simulink model "Phasor_load"  (R2024a)
settings: Solver=ode1  StartTime=0.0  StopTime=simtime  FixedStep=Ts  RelTol=1e-3
values from neighbouring files (symbols this model uses):
  c0 = c0_hawk    (= 6.37282e-09)    [EMT_Phasor_parameters.m]
  c1 = c1_hawk    (= 8.76156e-09)    [EMT_Phasor_parameters.m]
  fg = 50    [EMT_Phasor_parameters.m]
  G1gen = 0.1245    [EMT_Phasor_parameters.m]
  G2gen = 0.30    (= 0.3)    [EMT_Phasor_parameters.m]
  G3gen = 0.20    (= 0.2)    [EMT_Phasor_parameters.m]
  G4sgen = 0.2078    [EMT_Phasor_parameters.m]
  G5gen = 0.20    (= 0.2)    [EMT_Phasor_parameters.m]
  G6gen = 0.2078    [EMT_Phasor_parameters.m]
  G6sgen = 0.20    (= 0.2)    [EMT_Phasor_parameters.m]
  G7gen = 0.518    [EMT_Phasor_parameters.m]
  Ihvpk = Ihv*sqrt(2)    [EMT_Phasor_parameters.m]
  l0 = l0_hawk    (= 0.00373)    [EMT_Phasor_parameters.m]
  l1 = l1_hawk    (= 0.00133)    [EMT_Phasor_parameters.m]
  L3dem = 0.10    (= 0.1)    [EMT_Phasor_parameters.m]
  L4dem = 0.30    (= 0.3)    [EMT_Phasor_parameters.m]
  L5dem = 0.35    [EMT_Phasor_parameters.m]
  L6dem = 0.15    [EMT_Phasor_parameters.m]
  L7dem = 0.10    (= 0.1)    [EMT_Phasor_parameters.m]
  Pr = Sr*PF    (= 550050000)    [EMT_Phasor_parameters.m]
  Qr = sqrt(Sr^2 - Pr^2)    [EMT_Phasor_parameters.m]
  r0 = r0_hawk    (= 0.44587)    [EMT_Phasor_parameters.m]
  r1 = r1_hawk    (= 0.12087)    [EMT_Phasor_parameters.m]
  Rtpu = Xtpu/40    (= 0.00375)    [EMT_Phasor_parameters.m]
  S1non = 400e6    (= 400000000)    [EMT_Phasor_parameters.m]
  S2non = 300e6    (= 300000000)    [EMT_Phasor_parameters.m]
  S3non = 200e6    (= 200000000)    [EMT_Phasor_parameters.m]
  S4snon = 200e6    (= 200000000)    [EMT_Phasor_parameters.m]
  S5non = 500e6    (= 500000000)    [EMT_Phasor_parameters.m]
  S6non = 400e6    (= 400000000)    [EMT_Phasor_parameters.m]
  S6snon = 200e6    (= 200000000)    [EMT_Phasor_parameters.m]
  S7non = 200e6    (= 200000000)    [EMT_Phasor_parameters.m]
  simtime = 5    [EMT_Phasor_parameters.m]
  tonvsc = 0.01    [EMT_Phasor_parameters.m]
  Ts = 150e-6    (= 0.00015)    [EMT_Phasor_parameters.m]
  Vhv = 220e3    (= 220000)    [EMT_Phasor_parameters.m]
  Vmv = 22e3    (= 22000)    [EMT_Phasor_parameters.m]
  wc1 = wsw1/10    (= 848.230016469)    [EMT_Phasor_parameters.m]
  wdc1 = wc1/10    (= 84.8230016469)    [EMT_Phasor_parameters.m]
  wpq1 = wc1/10    (= 84.8230016469)    [EMT_Phasor_parameters.m]
  wsw1 = ksw1*2*pi*fg    (= 8482.30016469)    [EMT_Phasor_parameters.m]
  Xtpu = 0.15    [EMT_Phasor_parameters.m]
undefined symbols (not defined in the file or in its folder): D11, Delta, Kf, r, theta0
libraries: simulink_extras x152, spsGroundLib x52, powerlib_meascontrol x52, pid_lib x40, spsCurrentMeasurementLib x39, spsVoltageMeasurementLib x33, simulink x32, eeGeneralControl x32, eeTransforms x24, powerlib x24, spsFirstOrderFilterLib x16, spsControlledCurrentSourceLib x12
(part 16 of 17)

== system Phasor_load/G6/VSC/VSC Control/Modulation/Phasor Quasi-EMT/V to I RL (+seq) ==
  note: d-q axis model of a 3-phase series R-L branch
  note: Using Laplace transform:
  note: Iq = (Vq1 - Vq2 - w*L*Id)/(R + s*L)
  note: Id = (Vd1 - Vd2 + w*L*Iq)/(R + s*L)
  note: V2
  note: ==========================================================================================
  note: V1
  note: Vq1 - Vq2 = [ R * Iq ] + [ L* w * Id ] + [ L * d/dt (Iq) ]
  note: where w = 2*pi*f
  note: I --->
  note: o--------| R |---| L |-------o
  note: Vd1 - Vd2 = [ R * Id ] - [ L* w * Iq ] + [ L * d/dt (Id) ]
  note: This subsystem converts the VSC output voltage in a current signal through an RL element
  Vdq1 : Inport
  Vdq2 : Inport  Port=2
  Cartesian to Polar : simulink_extras/Transformations/Cartesian to Polar
  Delay : Delay  DelayLength=1
  Demux : Demux  Outputs=2
  Mux : Mux  Inputs=2
  Polar to Cartesian : simulink_extras/Transformations/Polar to Cartesian
  R_choke1 : Gain  Gain=w*L  SaturateOnIntegerOverflow=on  OutDataTypeStr=Inherit: Same as input  ParamDataTypeStr=Inherit: Same as input
  R_choke2 : Gain  Gain=[1 -1]  SaturateOnIntegerOverflow=on  OutDataTypeStr=Inherit: Same as input  ParamDataTypeStr=Inherit: Same as input
  Saturation : Saturate  UpperLimit=Imax  LowerLimit=0
  Selector : Selector  InputPortWidth=2  IndexOptions=Index vector (dialog)  Indices=[2 1]  OutputSizes=1
  Sum : Sum  Inputs=+-+  SaturateOnIntegerOverflow=on
  Transfer Fcn (with initial outputs) : simulink_extras/Additional Linear/Transfer Fcn (with initial outputs)  N=[1]  D=[L R]  Y0=0  U0=0
  Transfer Fcn (with initial outputs)1 : simulink_extras/Additional Linear/Transfer Fcn (with initial outputs)  N=[1]  D=[L R]  Y0=0  U0=0
  idIq : Outport  VectorParamsAs1DForOutWhenUnconnected=off
  wires:
  Selector/1 -> R_choke1/1
  Vdq1/1 -> Sum/1
  R_choke1/1 -> R_choke2/1
  Sum/1 -> Demux/1
  Demux/1 -> Transfer Fcn (with initial outputs)/1
  Demux/2 -> Transfer Fcn (with initial outputs)1/1
  Polar to Cartesian/1 -> Mux/1
  Polar to Cartesian/2 -> Mux/2
  Cartesian to Polar/2 -> Polar to Cartesian/2
  Mux/1 -> Delay/1, idIq/1
  R_choke2/1 -> Sum/3
  Transfer Fcn (with initial outputs)/1 -> Cartesian to Polar/1
  Transfer Fcn (with initial outputs)1/1 -> Cartesian to Polar/2
  Vdq2/1 -> Sum/2
  Cartesian to Polar/1 -> Saturation/1
  Saturation/1 -> Polar to Cartesian/1
  Delay/1 -> Selector/1

== system Phasor_load/G6/VSC/VSC Control/Modulation/Phasor Quasi-EMT/V to I RL (- seq) ==
  note: d-q axis model of a 3-phase series R-L branch
  note: Using Laplace transform:
  note: Iq = (Vq1 - Vq2 - w*L*Id)/(R + s*L)
  note: Id = (Vd1 - Vd2 + w*L*Iq)/(R + s*L)
  note: V2
  note: ==========================================================================================
  note: V1
  note: Vq1 - Vq2 = [ R * Iq ] + [ L* w * Id ] + [ L * d/dt (Iq) ]
  note: where w = 2*pi*f
  note: I --->
  note: o--------| R |---| L |-------o
  note: Vd1 - Vd2 = [ R * Id ] - [ L* w * Iq ] + [ L * d/dt (Id) ]
  note: This subsystem converts the VSC output voltage in a current signal through an RL element
  Vdq1 : Inport
  Vdq2 : Inport  Port=2
  Cartesian to Polar : simulink_extras/Transformations/Cartesian to Polar
  Delay : Delay  DelayLength=1
  Demux : Demux  Outputs=2
  Mux : Mux  Inputs=2
  Polar to Cartesian : simulink_extras/Transformations/Polar to Cartesian
  R_choke1 : Gain  Gain=w*L  SaturateOnIntegerOverflow=on  OutDataTypeStr=Inherit: Same as input  ParamDataTypeStr=Inherit: Same as input
  R_choke2 : Gain  Gain=[-1 1]  SaturateOnIntegerOverflow=on  OutDataTypeStr=Inherit: Same as input  ParamDataTypeStr=Inherit: Same as input
  Saturation : Saturate  UpperLimit=Imax  LowerLimit=0
  Selector : Selector  InputPortWidth=2  IndexOptions=Index vector (dialog)  Indices=[2 1]  OutputSizes=1
  Sum : Sum  Inputs=+-+  SaturateOnIntegerOverflow=on
  Transfer Fcn (with initial outputs) : simulink_extras/Additional Linear/Transfer Fcn (with initial outputs)  N=[1]  D=[L R]  Y0=0  U0=0
  Transfer Fcn (with initial outputs)1 : simulink_extras/Additional Linear/Transfer Fcn (with initial outputs)  N=[1]  D=[L R]  Y0=0  U0=0
  idIq : Outport  VectorParamsAs1DForOutWhenUnconnected=off
  wires:
  Selector/1 -> R_choke1/1
  Vdq1/1 -> Sum/1
  R_choke1/1 -> R_choke2/1
  Sum/1 -> Demux/1
  Demux/1 -> Transfer Fcn (with initial outputs)/1
  Demux/2 -> Transfer Fcn (with initial outputs)1/1
  Polar to Cartesian/1 -> Mux/1
  Polar to Cartesian/2 -> Mux/2
  Cartesian to Polar/2 -> Polar to Cartesian/2
  Mux/1 -> Delay/1, idIq/1
  R_choke2/1 -> Sum/3
  Transfer Fcn (with initial outputs)/1 -> Cartesian to Polar/1
  Transfer Fcn (with initial outputs)1/1 -> Cartesian to Polar/2
  Vdq2/1 -> Sum/2
  Cartesian to Polar/1 -> Saturation/1
  Saturation/1 -> Polar to Cartesian/1
  Delay/1 -> Selector/1

== system Phasor_load/G2/VSC/VSC Control/Control loops/Phasor I 1st/Outer-loop/Power calculation ==
  note: AC power calculation using symmetrical components in dq axis
  note: Pavgp = 3/2*(vqp*iqp + vdp*idp) and Qavgp = 3/2*(vqp*idp-vdp*iqp)
  note: P = Pavg + Pc2*cos(2wt) + Ps2*sin(2wt) ---> Pavg = Pavgp + Pavgn
  note: Q = Qavg + Qc2*cos(2wt) + Qs2*sin(2wt) ---> Qavg = Qavgp + Qavgn
  note: Pavgn = 3/2*(vqn*iqn + vdn*idn) and Qavgn = 3/2*(vqn*idn-vdn*iqn)
  vq+ : Inport
  vd+ : Inport  Port=2
  iq+ : Inport  Port=3
  id+ : Inport  Port=4
  vq- : Inport  Port=5
  vd- : Inport  Port=6
  iq- : Inport  Port=7
  id- : Inport  Port=8
  Gain : Gain  Gain=3/2
  Gain1 : Gain  Gain=3/2
  Gain2 : Gain  Gain=-1
  Gain3 : Gain  Gain=-1
  Mux{,1..3} (4 alike) : Mux  Inputs=2
  Product{,1..3} (4 alike) : Product
  Sum1 : Sum
  Sum2 : Sum
  Sum8 : Sum
  PQ : Outport
  wires:
  Sum8/1 -> Gain/1
  Gain2/1 -> Mux2/2
  Mux2/1 -> Product2/2
  Product2/1 -> Sum8/2
  Mux/1 -> Product/2
  Product/1 -> Sum8/1
  iq+/1 -> [iqp]
  [iqp] -> Gain2/1, Mux/1
  id+/1 -> [idp]
  [idp] -> Mux2/1, Mux/2
  vq+/1 -> [vqp]
  [vqp] -> Product/1
  vd+/1 -> [vdp]
  [vdp] -> Product2/1
  Gain/1 -> Sum1/1
  Sum1/1 -> PQ/1
  Gain3/1 -> Mux3/2
  Mux1/1 -> Product1/2
  Product3/1 -> Sum2/2
  Product1/1 -> Sum2/1
  [vdn] -> Product3/1
  Mux3/1 -> Product3/2
  [vqn] -> Product1/1
  Sum2/1 -> Gain1/1
  [iqn] -> Gain3/1, Mux1/1
  [idn] -> Mux3/1, Mux1/2
  vq-/1 -> [vqn]
  vd-/1 -> [vdn]
  iq-/1 -> [iqn]
  id-/1 -> [idn]
  Gain1/1 -> Sum1/2

== system Phasor_load/G2/VSC/VSC Control/Control loops/Phasor I ref/Outer-loop/Power calculation ==
  note: Pavgn = 3/2*(vqn*iqn + vdn*idn) and Qavgn = 3/2*(vqn*idn-vdn*iqn)
  note: Q = Qavg + Qc2*cos(2wt) + Qs2*sin(2wt) ---> Qavg = Qavgp + Qavgn
  note: P = Pavg + Pc2*cos(2wt) + Ps2*sin(2wt) ---> Pavg = Pavgp + Pavgn
  note: Pavgp = 3/2*(vqp*iqp + vdp*idp) and Qavgp = 3/2*(vqp*idp-vdp*iqp)
  note: AC power calculation using symmetrical components in dq axis
  vq+ : Inport
  vd+ : Inport  Port=2
  iq+ : Inport  Port=3
  id+ : Inport  Port=4
  vq- : Inport  Port=5
  vd- : Inport  Port=6
  iq- : Inport  Port=7
  id- : Inport  Port=8
  Gain : Gain  Gain=3/2
  Gain1 : Gain  Gain=3/2
  Gain2 : Gain  Gain=-1
  Gain3 : Gain  Gain=-1
  Mux{,1..3} (4 alike) : Mux  Inputs=2
  Product{,1..3} (4 alike) : Product
  Sum1 : Sum
  Sum2 : Sum
  Sum8 : Sum
  PQ : Outport
  wires:
  Gain1/1 -> Sum1/2
  id-/1 -> [idn]
  iq-/1 -> [iqn]
  vd-/1 -> [vdn]
  vq-/1 -> [vqn]
  [idn] -> Mux1/2, Mux3/1
  [iqn] -> Mux1/1, Gain3/1
  Sum2/1 -> Gain1/1
  [vqn] -> Product1/1
  Mux3/1 -> Product3/2
  [vdn] -> Product3/1
  Product1/1 -> Sum2/1
  Product3/1 -> Sum2/2
  Mux1/1 -> Product1/2
  Gain3/1 -> Mux3/2
  Sum1/1 -> PQ/1
  Gain/1 -> Sum1/1
  [vdp] -> Product2/1
  vd+/1 -> [vdp]
  [vqp] -> Product/1
  vq+/1 -> [vqp]
  [idp] -> Mux/2, Mux2/1
  id+/1 -> [idp]
  [iqp] -> Mux/1, Gain2/1
  iq+/1 -> [iqp]
  Product/1 -> Sum8/1
  Mux/1 -> Product/2
  Product2/1 -> Sum8/2
  Mux2/1 -> Product2/2
  Gain2/1 -> Mux2/2
  Sum8/1 -> Gain/1

== system Phasor_load/G2/VSC/VSC Control/Control loops/Phasor PQ 1st/Outer-loop/Power calculation ==
  note: AC power calculation using symmetrical components in dq axis
  note: Pavgp = 3/2*(vqp*iqp + vdp*idp) and Qavgp = 3/2*(vqp*idp-vdp*iqp)
  note: P = Pavg + Pc2*cos(2wt) + Ps2*sin(2wt) ---> Pavg = Pavgp + Pavgn
  note: Q = Qavg + Qc2*cos(2wt) + Qs2*sin(2wt) ---> Qavg = Qavgp + Qavgn
  note: Pavgn = 3/2*(vqn*iqn + vdn*idn) and Qavgn = 3/2*(vqn*idn-vdn*iqn)
  vq+ : Inport
  vd+ : Inport  Port=2
  iq+ : Inport  Port=3
  id+ : Inport  Port=4
  vq- : Inport  Port=5
  vd- : Inport  Port=6
  iq- : Inport  Port=7
  id- : Inport  Port=8
  Gain : Gain  Gain=3/2
  Gain1 : Gain  Gain=3/2
  Gain2 : Gain  Gain=-1
  Gain3 : Gain  Gain=-1
  Mux{,1..3} (4 alike) : Mux  Inputs=2
  Product{,1..3} (4 alike) : Product
  Sum1 : Sum
  Sum2 : Sum
  Sum8 : Sum
  PQ : Outport
  wires:
  Sum8/1 -> Gain/1
  Gain2/1 -> Mux2/2
  Mux2/1 -> Product2/2
  Product2/1 -> Sum8/2
  Mux/1 -> Product/2
  Product/1 -> Sum8/1
  iq+/1 -> [iqp]
  [iqp] -> Gain2/1, Mux/1
  id+/1 -> [idp]
  [idp] -> Mux2/1, Mux/2
  vq+/1 -> [vqp]
  [vqp] -> Product/1
  vd+/1 -> [vdp]
  [vdp] -> Product2/1
  Gain/1 -> Sum1/1
  Sum1/1 -> PQ/1
  Gain3/1 -> Mux3/2
  Mux1/1 -> Product1/2
  Product3/1 -> Sum2/2
  Product1/1 -> Sum2/1
  [vdn] -> Product3/1
  Mux3/1 -> Product3/2
  [vqn] -> Product1/1
  Sum2/1 -> Gain1/1
  [iqn] -> Gain3/1, Mux1/1
  [idn] -> Mux3/1, Mux1/2
  vq-/1 -> [vqn]
  vd-/1 -> [vdn]
  iq-/1 -> [iqn]
  id-/1 -> [idn]
  Gain1/1 -> Sum1/2

== system Phasor_load/G2/VSC/VSC Control/Control loops/SW, EMT AVG, Phasor Quasi-EMT/Outer-loop/Power calculation ==
  note: AC power calculation using symmetrical components in dq axis
  note: Pavgp = 3/2*(vqp*iqp + vdp*idp) and Qavgp = 3/2*(vqp*idp-vdp*iqp)
  note: P = Pavg + Pc2*cos(2wt) + Ps2*sin(2wt) ---> Pavg = Pavgp + Pavgn
  note: Q = Qavg + Qc2*cos(2wt) + Qs2*sin(2wt) ---> Qavg = Qavgp + Qavgn
  note: Pavgn = 3/2*(vqn*iqn + vdn*idn) and Qavgn = 3/2*(vqn*idn-vdn*iqn)
  vq+ : Inport
  vd+ : Inport  Port=2
  iq+ : Inport  Port=3
  id+ : Inport  Port=4
  vq- : Inport  Port=5
  vd- : Inport  Port=6
  iq- : Inport  Port=7
  id- : Inport  Port=8
  Gain : Gain  Gain=3/2
  Gain1 : Gain  Gain=3/2
  Gain2 : Gain  Gain=-1
  Gain3 : Gain  Gain=-1
  Mux{,1..3} (4 alike) : Mux  Inputs=2
  Product{,1..3} (4 alike) : Product
  Sum1 : Sum
  Sum2 : Sum
  Sum8 : Sum
  PQ : Outport
  wires:
  Sum8/1 -> Gain/1
  Gain2/1 -> Mux2/2
  Mux2/1 -> Product2/2
  Product2/1 -> Sum8/2
  Mux/1 -> Product/2
  Product/1 -> Sum8/1
  iq+/1 -> [iqp]
  [iqp] -> Gain2/1, Mux/1
  id+/1 -> [idp]
  [idp] -> Mux2/1, Mux/2
  vq+/1 -> [vqp]
  [vqp] -> Product/1
  vd+/1 -> [vdp]
  [vdp] -> Product2/1
  Gain/1 -> Sum1/1
  Sum1/1 -> PQ/1
  Gain3/1 -> Mux3/2
  Mux1/1 -> Product1/2
  Product3/1 -> Sum2/2
  Product1/1 -> Sum2/1
  [vdn] -> Product3/1
  Mux3/1 -> Product3/2
  [vqn] -> Product1/1
  Sum2/1 -> Gain1/1
  [iqn] -> Gain3/1, Mux1/1
  [idn] -> Mux3/1, Mux1/2
  vq-/1 -> [vqn]
  vd-/1 -> [vdn]
  iq-/1 -> [iqn]
  id-/1 -> [idn]
  Gain1/1 -> Sum1/2

== system Phasor_load/G2/VSC/VSC Control/Measurements/EMT/PLL aligned with positive-sequence/Notch filter ==
  In : Inport
  Discrete Transfer Fcn : DiscreteTransferFcn  Numerator=[1, -2*cos(theta0), 1]  Denominator="[1, -2*cos(theta0)*r,  r^2]"
  Gain7 : Gain  Gain=Kf
  Out : Outport
  wires:
  Gain7/1 -> Discrete Transfer Fcn/1
  Discrete Transfer Fcn/1 -> Out/1
  In/1 -> Gain7/1

== system Phasor_load/G2/VSC/VSC Control/Measurements/EMT/PLL aligned with positive-sequence/Park transform ==
  note: Park transform (q axis leading)
  abc : Inport
  theta : Inport  Port=2
  0 : Fcn  Expr=1/3*(u(1) + u(2) + u(3))
  Mux2 : Mux  Inputs=2
  Mux3 : Mux  Inputs=3
  d : Fcn  Expr=2/3*(u(1)*sin(u(4)) + u(2)*sin(u(4) - (2*pi)/3) + u(3)*sin(u(4) + (2*pi)/3))
  q : Fcn  Expr=2/3*(u(1)*cos(u(4)) + u(2)*cos(u(4) - (2*pi)/3) + u(3)*cos(u(4) + (2*pi)/3))
  qd0 : Outport  VectorParamsAs1DForOutWhenUnconnected=off
  wires:
  q/1 -> Mux3/1
  Mux2/1 -> q/1, 0/1, d/1
  0/1 -> Mux3/3
  d/1 -> Mux3/2
  theta/1 -> Mux2/2
  abc/1 -> Mux2/1
  Mux3/1 -> qd0/1

== system Phasor_load/G2/VSC/VSC Control/Measurements/EMT/PLL aligned with positive-sequence/Phase-sequence separation ==
  note: Phase-sequence separation based on
      | Delayed Signal Cancellation (DSC) method
  abc : Inport
  Theta : Inport  Port=2
  Complex to Real-Imag1 : ComplexToRealImag
  Complex to Real-Imag2 : ComplexToRealImag
  Complex to Real-Imag3 : ComplexToRealImag
  Constant : Constant  Value=negseq_en
  Demux3 : Demux  Outputs=3
  Exp2 : Math  OutputSignalType=complex
  Exp3 : Math  OutputSignalType=complex
  Gain1 : Gain  Gain=1/2
  Gain4 : Gain  Gain=-1i
  Gain5 : Gain  Gain=1i
  Gain6 : Gain  Gain=1/2
  Gain7 : Gain  Gain=1i
  NOT : Logic  Operator=NOT  IconShape=distinctive  AllPortsSameDT=off  OutDataTypeStr=boolean
  Product3 : Product
  Product4 : Product
  Real-Imag to Complex : RealImagToComplex
  Real-Imag to Complex1 : RealImagToComplex
  Sum1 : Sum  Inputs=|++
  Sum2 : Sum  Inputs=-+|
  Switch : Switch  Criteria=u2 ~= 0  SaturateOnIntegerOverflow=off  InputSameDT=off
  Terminator3 : Terminator
  Transport Delay2 : TransportDelay  DelayTime=1/4*(1/50)
  Transport Delay3 : TransportDelay  DelayTime=1/4*(1/50)
  abc to Alpha-Beta-Zero : powerlib_meascontrol/Transformations/abc to Alpha-Beta-Zero
  q+ : Outport
  d+ : Outport  Port=2
  q- : Outport  Port=3
  d- : Outport  Port=4
  wires:
  NOT/1 -> Switch/2
  Constant/1 -> NOT/1
  Switch/1 -> Product3/1
  Gain6/1 -> Switch/3
  Sum2/1 -> Gain1/1
  Transport Delay2/1 -> Real-Imag to Complex1/1
  Demux3/1 -> Real-Imag to Complex/1
  Complex to Real-Imag1/2 -> Transport Delay3/1
  Gain1/1 -> Product4/2
  Real-Imag to Complex/1 -> Complex to Real-Imag1/1, Sum2/2, Sum1/1, Switch/1
  Complex to Real-Imag3/1 -> d-/1
  Real-Imag to Complex1/1 -> Gain5/1
  Complex to Real-Imag1/1 -> Transport Delay2/1
  Transport Delay3/1 -> Real-Imag to Complex1/2
  Demux3/2 -> Real-Imag to Complex/2
  Product3/1 -> Complex to Real-Imag2/1
  Product4/1 -> Complex to Real-Imag3/1
  abc to Alpha-Beta-Zero/1 -> Demux3/1
  abc/1 -> abc to Alpha-Beta-Zero/1
  Exp3/1 -> Product4/1
  Complex to Real-Imag3/2 -> q-/1
  Complex to Real-Imag2/2 -> q+/1
  Demux3/3 -> Terminator3/1
  Sum1/1 -> Gain6/1
  Gain5/1 -> Sum2/1, Sum1/2
  Exp2/1 -> Product3/2
  Gain4/1 -> Exp2/1
  Theta/1 -> Gain4/1, Gain7/1
  Gain7/1 -> Exp3/1
  Complex to Real-Imag2/1 -> d+/1

== system Phasor_load/G2/VSC/VSC Control/Measurements/EMT/PLL aligned with positive-sequence/Subsystem ==
  note: PI controller with reset port and initial conditions restored after reset or after maximum/minimum values are reached
  in : Inport
  Reset : Inport  Port=2
  Compare To Constant2 : simulink/Logic and Bit Operations/Compare To Constant  relop=~=  const=0  OutDataTypeStr=boolean
  Constant2 : Constant  Value=2*pi*fg
  Gain : Gain  Gain=kp_pll
  Gain1 : Gain  Gain=kp_pll/tau_pll
  Integrator Limited : Integrator  ExternalReset=level  InitialCondition=2*pi*fg  UpperSaturationLimit=10.1*2*pi*fg  LowerSaturationLimit=0.09*2*pi*fg  ShowSaturationPort=on
  Memory1 : Memory
  NOT : Logic  Operator=NOT  IconShape=distinctive  AllPortsSameDT=off  OutDataTypeStr=boolean
  OR2 : Logic  Operator=OR  IconShape=distinctive  AllPortsSameDT=off  OutDataTypeStr=boolean
  Product : Product
  Sum : Sum
  Switch1 : Switch  SaturateOnIntegerOverflow=off  InputSameDT=off
  w : Outport
  wires:
  Switch1/1 -> w/1
  Product/1 -> Gain1/1, Gain/1
  Gain1/1 -> Integrator Limited/1
  Integrator Limited/2 -> Compare To Constant2/1, Switch1/2
  Compare To Constant2/1 -> Memory1/1
  OR2/1 -> Integrator Limited/2, NOT/1
  Constant2/1 -> Switch1/3
  Memory1/1 -> OR2/1
  Reset/1 -> OR2/2
  Gain/1 -> Sum/1
  Integrator Limited/1 -> Sum/2
  Sum/1 -> Switch1/1
  in/1 -> Product/1
  NOT/1 -> Product/2

== system Phasor_load/G2/VSC/VSC Control/Modulation/Phasor I and Phasor PQ/RL time constant/Corrects delay ==
  Clock : Clock
  Gain : Gain  Gain=(2*pi*fg)
  Memory : Memory
  Sum : Sum  Inputs=|+-
  dphi : Outport
  wires:
  Gain/1 -> dphi/1
  Sum/1 -> Gain/1  "Ts"
  Memory/1 -> Sum/2
  Clock/1 -> Sum/1, Memory/1

== system Phasor_load/G3/VSC/VSC Control/Control loops/Phasor I 1st/Outer-loop/Power calculation ==
  note: AC power calculation using symmetrical components in dq axis
  note: Pavgp = 3/2*(vqp*iqp + vdp*idp) and Qavgp = 3/2*(vqp*idp-vdp*iqp)
  note: P = Pavg + Pc2*cos(2wt) + Ps2*sin(2wt) ---> Pavg = Pavgp + Pavgn
  note: Q = Qavg + Qc2*cos(2wt) + Qs2*sin(2wt) ---> Qavg = Qavgp + Qavgn
  note: Pavgn = 3/2*(vqn*iqn + vdn*idn) and Qavgn = 3/2*(vqn*idn-vdn*iqn)
  vq+ : Inport
  vd+ : Inport  Port=2
  iq+ : Inport  Port=3
  id+ : Inport  Port=4
  vq- : Inport  Port=5
  vd- : Inport  Port=6
  iq- : Inport  Port=7
  id- : Inport  Port=8
  Gain : Gain  Gain=3/2
  Gain1 : Gain  Gain=3/2
  Gain2 : Gain  Gain=-1
  Gain3 : Gain  Gain=-1
  Mux{,1..3} (4 alike) : Mux  Inputs=2
  Product{,1..3} (4 alike) : Product
  Sum1 : Sum
  Sum2 : Sum
  Sum8 : Sum
  PQ : Outport
  wires:
  Sum8/1 -> Gain/1
  Gain2/1 -> Mux2/2
  Mux2/1 -> Product2/2
  Product2/1 -> Sum8/2
  Mux/1 -> Product/2
  Product/1 -> Sum8/1
  iq+/1 -> [iqp]
  [iqp] -> Gain2/1, Mux/1
  id+/1 -> [idp]
  [idp] -> Mux2/1, Mux/2
  vq+/1 -> [vqp]
  [vqp] -> Product/1
  vd+/1 -> [vdp]
  [vdp] -> Product2/1
  Gain/1 -> Sum1/1
  Sum1/1 -> PQ/1
  Gain3/1 -> Mux3/2
  Mux1/1 -> Product1/2
  Product3/1 -> Sum2/2
  Product1/1 -> Sum2/1
  [vdn] -> Product3/1
  Mux3/1 -> Product3/2
  [vqn] -> Product1/1
  Sum2/1 -> Gain1/1
  [iqn] -> Gain3/1, Mux1/1
  [idn] -> Mux3/1, Mux1/2
  vq-/1 -> [vqn]
  vd-/1 -> [vdn]
  iq-/1 -> [iqn]
  id-/1 -> [idn]
  Gain1/1 -> Sum1/2

== system Phasor_load/G3/VSC/VSC Control/Control loops/Phasor I ref/Outer-loop/Power calculation ==
  note: Pavgn = 3/2*(vqn*iqn + vdn*idn) and Qavgn = 3/2*(vqn*idn-vdn*iqn)
  note: Q = Qavg + Qc2*cos(2wt) + Qs2*sin(2wt) ---> Qavg = Qavgp + Qavgn
  note: P = Pavg + Pc2*cos(2wt) + Ps2*sin(2wt) ---> Pavg = Pavgp + Pavgn
  note: Pavgp = 3/2*(vqp*iqp + vdp*idp) and Qavgp = 3/2*(vqp*idp-vdp*iqp)
  note: AC power calculation using symmetrical components in dq axis
  vq+ : Inport
  vd+ : Inport  Port=2
  iq+ : Inport  Port=3
  id+ : Inport  Port=4
  vq- : Inport  Port=5
  vd- : Inport  Port=6
  iq- : Inport  Port=7
  id- : Inport  Port=8
  Gain : Gain  Gain=3/2
  Gain1 : Gain  Gain=3/2
  Gain2 : Gain  Gain=-1
  Gain3 : Gain  Gain=-1
  Mux{,1..3} (4 alike) : Mux  Inputs=2
  Product{,1..3} (4 alike) : Product
  Sum1 : Sum
  Sum2 : Sum
  Sum8 : Sum
  PQ : Outport
  wires:
  Gain1/1 -> Sum1/2
  id-/1 -> [idn]
  iq-/1 -> [iqn]
  vd-/1 -> [vdn]
  vq-/1 -> [vqn]
  [idn] -> Mux1/2, Mux3/1
  [iqn] -> Mux1/1, Gain3/1
  Sum2/1 -> Gain1/1
  [vqn] -> Product1/1
  Mux3/1 -> Product3/2
  [vdn] -> Product3/1
  Product1/1 -> Sum2/1
  Product3/1 -> Sum2/2
  Mux1/1 -> Product1/2
  Gain3/1 -> Mux3/2
  Sum1/1 -> PQ/1
  Gain/1 -> Sum1/1
  [vdp] -> Product2/1
  vd+/1 -> [vdp]
  [vqp] -> Product/1
  vq+/1 -> [vqp]
  [idp] -> Mux/2, Mux2/1
  id+/1 -> [idp]
  [iqp] -> Mux/1, Gain2/1
  iq+/1 -> [iqp]
  Product/1 -> Sum8/1
  Mux/1 -> Product/2
  Product2/1 -> Sum8/2
  Mux2/1 -> Product2/2
  Gain2/1 -> Mux2/2
  Sum8/1 -> Gain/1

== system Phasor_load/G3/VSC/VSC Control/Control loops/Phasor PQ 1st/Outer-loop/Power calculation ==
  note: AC power calculation using symmetrical components in dq axis
  note: Pavgp = 3/2*(vqp*iqp + vdp*idp) and Qavgp = 3/2*(vqp*idp-vdp*iqp)
  note: P = Pavg + Pc2*cos(2wt) + Ps2*sin(2wt) ---> Pavg = Pavgp + Pavgn
  note: Q = Qavg + Qc2*cos(2wt) + Qs2*sin(2wt) ---> Qavg = Qavgp + Qavgn
  note: Pavgn = 3/2*(vqn*iqn + vdn*idn) and Qavgn = 3/2*(vqn*idn-vdn*iqn)
  vq+ : Inport
  vd+ : Inport  Port=2
  iq+ : Inport  Port=3
  id+ : Inport  Port=4
  vq- : Inport  Port=5
  vd- : Inport  Port=6
  iq- : Inport  Port=7
  id- : Inport  Port=8
  Gain : Gain  Gain=3/2
  Gain1 : Gain  Gain=3/2
  Gain2 : Gain  Gain=-1
  Gain3 : Gain  Gain=-1
  Mux{,1..3} (4 alike) : Mux  Inputs=2
  Product{,1..3} (4 alike) : Product
  Sum1 : Sum
  Sum2 : Sum
  Sum8 : Sum
  PQ : Outport
  wires:
  Sum8/1 -> Gain/1
  Gain2/1 -> Mux2/2
  Mux2/1 -> Product2/2
  Product2/1 -> Sum8/2
  Mux/1 -> Product/2
  Product/1 -> Sum8/1
  iq+/1 -> [iqp]
  [iqp] -> Gain2/1, Mux/1
  id+/1 -> [idp]
  [idp] -> Mux2/1, Mux/2
  vq+/1 -> [vqp]
  [vqp] -> Product/1
  vd+/1 -> [vdp]
  [vdp] -> Product2/1
  Gain/1 -> Sum1/1
  Sum1/1 -> PQ/1
  Gain3/1 -> Mux3/2
  Mux1/1 -> Product1/2
  Product3/1 -> Sum2/2
  Product1/1 -> Sum2/1
  [vdn] -> Product3/1
  Mux3/1 -> Product3/2
  [vqn] -> Product1/1
  Sum2/1 -> Gain1/1
  [iqn] -> Gain3/1, Mux1/1
  [idn] -> Mux3/1, Mux1/2
  vq-/1 -> [vqn]
  vd-/1 -> [vdn]
  iq-/1 -> [iqn]
  id-/1 -> [idn]
  Gain1/1 -> Sum1/2

== system Phasor_load/G3/VSC/VSC Control/Control loops/SW, EMT AVG, Phasor Quasi-EMT/Outer-loop/Power calculation ==
  note: AC power calculation using symmetrical components in dq axis
  note: Pavgp = 3/2*(vqp*iqp + vdp*idp) and Qavgp = 3/2*(vqp*idp-vdp*iqp)
  note: P = Pavg + Pc2*cos(2wt) + Ps2*sin(2wt) ---> Pavg = Pavgp + Pavgn
  note: Q = Qavg + Qc2*cos(2wt) + Qs2*sin(2wt) ---> Qavg = Qavgp + Qavgn
  note: Pavgn = 3/2*(vqn*iqn + vdn*idn) and Qavgn = 3/2*(vqn*idn-vdn*iqn)
  vq+ : Inport
  vd+ : Inport  Port=2
  iq+ : Inport  Port=3
  id+ : Inport  Port=4
  vq- : Inport  Port=5
  vd- : Inport  Port=6
  iq- : Inport  Port=7
  id- : Inport  Port=8
  Gain : Gain  Gain=3/2
  Gain1 : Gain  Gain=3/2
  Gain2 : Gain  Gain=-1
  Gain3 : Gain  Gain=-1
  Mux{,1..3} (4 alike) : Mux  Inputs=2
  Product{,1..3} (4 alike) : Product
  Sum1 : Sum
  Sum2 : Sum
  Sum8 : Sum
  PQ : Outport
  wires:
  Sum8/1 -> Gain/1
  Gain2/1 -> Mux2/2
  Mux2/1 -> Product2/2
  Product2/1 -> Sum8/2
  Mux/1 -> Product/2
  Product/1 -> Sum8/1
  iq+/1 -> [iqp]
  [iqp] -> Gain2/1, Mux/1
  id+/1 -> [idp]
  [idp] -> Mux2/1, Mux/2
  vq+/1 -> [vqp]
  [vqp] -> Product/1
  vd+/1 -> [vdp]
  [vdp] -> Product2/1
  Gain/1 -> Sum1/1
  Sum1/1 -> PQ/1
  Gain3/1 -> Mux3/2
  Mux1/1 -> Product1/2
  Product3/1 -> Sum2/2
  Product1/1 -> Sum2/1
  [vdn] -> Product3/1
  Mux3/1 -> Product3/2
  [vqn] -> Product1/1
  Sum2/1 -> Gain1/1
  [iqn] -> Gain3/1, Mux1/1
  [idn] -> Mux3/1, Mux1/2
  vq-/1 -> [vqn]
  vd-/1 -> [vdn]
  iq-/1 -> [iqn]
  id-/1 -> [idn]
  Gain1/1 -> Sum1/2

== system Phasor_load/G3/VSC/VSC Control/Measurements/EMT/PLL aligned with positive-sequence/Notch filter ==
  In : Inport
  Discrete Transfer Fcn : DiscreteTransferFcn  Numerator=[1, -2*cos(theta0), 1]  Denominator="[1, -2*cos(theta0)*r,  r^2]"
  Gain7 : Gain  Gain=Kf
  Out : Outport
  wires:
  Gain7/1 -> Discrete Transfer Fcn/1
  Discrete Transfer Fcn/1 -> Out/1
  In/1 -> Gain7/1

== system Phasor_load/G3/VSC/VSC Control/Measurements/EMT/PLL aligned with positive-sequence/Park transform ==
  note: Park transform (q axis leading)
  abc : Inport
  theta : Inport  Port=2
  0 : Fcn  Expr=1/3*(u(1) + u(2) + u(3))
  Mux2 : Mux  Inputs=2
  Mux3 : Mux  Inputs=3
  d : Fcn  Expr=2/3*(u(1)*sin(u(4)) + u(2)*sin(u(4) - (2*pi)/3) + u(3)*sin(u(4) + (2*pi)/3))
  q : Fcn  Expr=2/3*(u(1)*cos(u(4)) + u(2)*cos(u(4) - (2*pi)/3) + u(3)*cos(u(4) + (2*pi)/3))
  qd0 : Outport  VectorParamsAs1DForOutWhenUnconnected=off
  wires:
  q/1 -> Mux3/1
  Mux2/1 -> q/1, 0/1, d/1
  0/1 -> Mux3/3
  d/1 -> Mux3/2
  theta/1 -> Mux2/2
  abc/1 -> Mux2/1
  Mux3/1 -> qd0/1

== system Phasor_load/G3/VSC/VSC Control/Measurements/EMT/PLL aligned with positive-sequence/Phase-sequence separation ==
  note: Phase-sequence separation based on
      | Delayed Signal Cancellation (DSC) method
  abc : Inport
  Theta : Inport  Port=2
  Complex to Real-Imag1 : ComplexToRealImag
  Complex to Real-Imag2 : ComplexToRealImag
  Complex to Real-Imag3 : ComplexToRealImag
  Constant : Constant  Value=negseq_en
  Demux3 : Demux  Outputs=3
  Exp2 : Math  OutputSignalType=complex
  Exp3 : Math  OutputSignalType=complex
  Gain1 : Gain  Gain=1/2
  Gain4 : Gain  Gain=-1i
  Gain5 : Gain  Gain=1i
  Gain6 : Gain  Gain=1/2
  Gain7 : Gain  Gain=1i
  NOT : Logic  Operator=NOT  IconShape=distinctive  AllPortsSameDT=off  OutDataTypeStr=boolean
  Product3 : Product
  Product4 : Product
  Real-Imag to Complex : RealImagToComplex
  Real-Imag to Complex1 : RealImagToComplex
  Sum1 : Sum  Inputs=|++
  Sum2 : Sum  Inputs=-+|
  Switch : Switch  Criteria=u2 ~= 0  SaturateOnIntegerOverflow=off  InputSameDT=off
  Terminator3 : Terminator
  Transport Delay2 : TransportDelay  DelayTime=1/4*(1/50)
  Transport Delay3 : TransportDelay  DelayTime=1/4*(1/50)
  abc to Alpha-Beta-Zero : powerlib_meascontrol/Transformations/abc to Alpha-Beta-Zero
  q+ : Outport
  d+ : Outport  Port=2
  q- : Outport  Port=3
  d- : Outport  Port=4
  wires:
  NOT/1 -> Switch/2
  Constant/1 -> NOT/1
  Switch/1 -> Product3/1
  Gain6/1 -> Switch/3
  Sum2/1 -> Gain1/1
  Transport Delay2/1 -> Real-Imag to Complex1/1
  Demux3/1 -> Real-Imag to Complex/1
  Complex to Real-Imag1/2 -> Transport Delay3/1
  Gain1/1 -> Product4/2
  Real-Imag to Complex/1 -> Complex to Real-Imag1/1, Sum2/2, Sum1/1, Switch/1
  Complex to Real-Imag3/1 -> d-/1
  Real-Imag to Complex1/1 -> Gain5/1
  Complex to Real-Imag1/1 -> Transport Delay2/1
  Transport Delay3/1 -> Real-Imag to Complex1/2
  Demux3/2 -> Real-Imag to Complex/2
  Product3/1 -> Complex to Real-Imag2/1
  Product4/1 -> Complex to Real-Imag3/1
  abc to Alpha-Beta-Zero/1 -> Demux3/1
  abc/1 -> abc to Alpha-Beta-Zero/1
  Exp3/1 -> Product4/1
  Complex to Real-Imag3/2 -> q-/1
  Complex to Real-Imag2/2 -> q+/1
  Demux3/3 -> Terminator3/1
  Sum1/1 -> Gain6/1
  Gain5/1 -> Sum2/1, Sum1/2
  Exp2/1 -> Product3/2
  Gain4/1 -> Exp2/1
  Theta/1 -> Gain4/1, Gain7/1
  Gain7/1 -> Exp3/1
  Complex to Real-Imag2/1 -> d+/1

== system Phasor_load/G3/VSC/VSC Control/Measurements/EMT/PLL aligned with positive-sequence/Subsystem ==
  note: PI controller with reset port and initial conditions restored after reset or after maximum/minimum values are reached
  in : Inport
  Reset : Inport  Port=2
  Compare To Constant2 : simulink/Logic and Bit Operations/Compare To Constant  relop=~=  const=0  OutDataTypeStr=boolean
  Constant2 : Constant  Value=2*pi*fg
  Gain : Gain  Gain=kp_pll
  Gain1 : Gain  Gain=kp_pll/tau_pll
  Integrator Limited : Integrator  ExternalReset=level  InitialCondition=2*pi*fg  UpperSaturationLimit=10.1*2*pi*fg  LowerSaturationLimit=0.09*2*pi*fg  ShowSaturationPort=on
  Memory1 : Memory
  NOT : Logic  Operator=NOT  IconShape=distinctive  AllPortsSameDT=off  OutDataTypeStr=boolean
  OR2 : Logic  Operator=OR  IconShape=distinctive  AllPortsSameDT=off  OutDataTypeStr=boolean
  Product : Product
  Sum : Sum
  Switch1 : Switch  SaturateOnIntegerOverflow=off  InputSameDT=off
  w : Outport
  wires:
  Switch1/1 -> w/1
  Product/1 -> Gain1/1, Gain/1
  Gain1/1 -> Integrator Limited/1
  Integrator Limited/2 -> Compare To Constant2/1, Switch1/2
  Compare To Constant2/1 -> Memory1/1
  OR2/1 -> Integrator Limited/2, NOT/1
  Constant2/1 -> Switch1/3
  Memory1/1 -> OR2/1
  Reset/1 -> OR2/2
  Gain/1 -> Sum/1
  Integrator Limited/1 -> Sum/2
  Sum/1 -> Switch1/1
  in/1 -> Product/1
  NOT/1 -> Product/2

== system Phasor_load/G3/VSC/VSC Control/Modulation/Phasor I and Phasor PQ/RL time constant/Corrects delay ==
  Clock : Clock
  Gain : Gain  Gain=(2*pi*fg)
  Memory : Memory
  Sum : Sum  Inputs=|+-
  dphi : Outport
  wires:
  Gain/1 -> dphi/1
  Sum/1 -> Gain/1  "Ts"
  Memory/1 -> Sum/2
  Clock/1 -> Sum/1, Memory/1

== system Phasor_load/G5/VSC/VSC Control/Control loops/Phasor I 1st/Outer-loop/Power calculation ==
  note: AC power calculation using symmetrical components in dq axis
  note: Pavgp = 3/2*(vqp*iqp + vdp*idp) and Qavgp = 3/2*(vqp*idp-vdp*iqp)
  note: P = Pavg + Pc2*cos(2wt) + Ps2*sin(2wt) ---> Pavg = Pavgp + Pavgn
  note: Q = Qavg + Qc2*cos(2wt) + Qs2*sin(2wt) ---> Qavg = Qavgp + Qavgn
  note: Pavgn = 3/2*(vqn*iqn + vdn*idn) and Qavgn = 3/2*(vqn*idn-vdn*iqn)
  vq+ : Inport
  vd+ : Inport  Port=2
  iq+ : Inport  Port=3
  id+ : Inport  Port=4
  vq- : Inport  Port=5
  vd- : Inport  Port=6
  iq- : Inport  Port=7
  id- : Inport  Port=8
  Gain : Gain  Gain=3/2
  Gain1 : Gain  Gain=3/2
  Gain2 : Gain  Gain=-1
  Gain3 : Gain  Gain=-1
  Mux{,1..3} (4 alike) : Mux  Inputs=2
  Product{,1..3} (4 alike) : Product
  Sum1 : Sum
  Sum2 : Sum
  Sum8 : Sum
  PQ : Outport
  wires:
  Sum8/1 -> Gain/1
  Gain2/1 -> Mux2/2
  Mux2/1 -> Product2/2
  Product2/1 -> Sum8/2
  Mux/1 -> Product/2
  Product/1 -> Sum8/1
  iq+/1 -> [iqp]
  [iqp] -> Gain2/1, Mux/1
  id+/1 -> [idp]
  [idp] -> Mux2/1, Mux/2
  vq+/1 -> [vqp]
  [vqp] -> Product/1
  vd+/1 -> [vdp]
  [vdp] -> Product2/1
  Gain/1 -> Sum1/1
  Sum1/1 -> PQ/1
  Gain3/1 -> Mux3/2
  Mux1/1 -> Product1/2
  Product3/1 -> Sum2/2
  Product1/1 -> Sum2/1
  [vdn] -> Product3/1
  Mux3/1 -> Product3/2
  [vqn] -> Product1/1
  Sum2/1 -> Gain1/1
  [iqn] -> Gain3/1, Mux1/1
  [idn] -> Mux3/1, Mux1/2
  vq-/1 -> [vqn]
  vd-/1 -> [vdn]
  iq-/1 -> [iqn]
  id-/1 -> [idn]
  Gain1/1 -> Sum1/2

== system Phasor_load/G5/VSC/VSC Control/Control loops/Phasor I ref/Outer-loop/Power calculation ==
  note: Pavgn = 3/2*(vqn*iqn + vdn*idn) and Qavgn = 3/2*(vqn*idn-vdn*iqn)
  note: Q = Qavg + Qc2*cos(2wt) + Qs2*sin(2wt) ---> Qavg = Qavgp + Qavgn
  note: P = Pavg + Pc2*cos(2wt) + Ps2*sin(2wt) ---> Pavg = Pavgp + Pavgn
  note: Pavgp = 3/2*(vqp*iqp + vdp*idp) and Qavgp = 3/2*(vqp*idp-vdp*iqp)
  note: AC power calculation using symmetrical components in dq axis
  vq+ : Inport
  vd+ : Inport  Port=2
  iq+ : Inport  Port=3
  id+ : Inport  Port=4
  vq- : Inport  Port=5
  vd- : Inport  Port=6
  iq- : Inport  Port=7
  id- : Inport  Port=8
  Gain : Gain  Gain=3/2
  Gain1 : Gain  Gain=3/2
  Gain2 : Gain  Gain=-1
  Gain3 : Gain  Gain=-1
  Mux{,1..3} (4 alike) : Mux  Inputs=2
  Product{,1..3} (4 alike) : Product
  Sum1 : Sum
  Sum2 : Sum
  Sum8 : Sum
  PQ : Outport
  wires:
  Gain1/1 -> Sum1/2
  id-/1 -> [idn]
  iq-/1 -> [iqn]
  vd-/1 -> [vdn]
  vq-/1 -> [vqn]
  [idn] -> Mux1/2, Mux3/1
  [iqn] -> Mux1/1, Gain3/1
  Sum2/1 -> Gain1/1
  [vqn] -> Product1/1
  Mux3/1 -> Product3/2
  [vdn] -> Product3/1
  Product1/1 -> Sum2/1
  Product3/1 -> Sum2/2
  Mux1/1 -> Product1/2
  Gain3/1 -> Mux3/2
  Sum1/1 -> PQ/1
  Gain/1 -> Sum1/1
  [vdp] -> Product2/1
  vd+/1 -> [vdp]
  [vqp] -> Product/1
  vq+/1 -> [vqp]
  [idp] -> Mux/2, Mux2/1
  id+/1 -> [idp]
  [iqp] -> Mux/1, Gain2/1
  iq+/1 -> [iqp]
  Product/1 -> Sum8/1
  Mux/1 -> Product/2
  Product2/1 -> Sum8/2
  Mux2/1 -> Product2/2
  Gain2/1 -> Mux2/2
  Sum8/1 -> Gain/1

== system Phasor_load/G5/VSC/VSC Control/Control loops/Phasor PQ 1st/Outer-loop/Power calculation ==
  note: AC power calculation using symmetrical components in dq axis
  note: Pavgp = 3/2*(vqp*iqp + vdp*idp) and Qavgp = 3/2*(vqp*idp-vdp*iqp)
  note: P = Pavg + Pc2*cos(2wt) + Ps2*sin(2wt) ---> Pavg = Pavgp + Pavgn
  note: Q = Qavg + Qc2*cos(2wt) + Qs2*sin(2wt) ---> Qavg = Qavgp + Qavgn
  note: Pavgn = 3/2*(vqn*iqn + vdn*idn) and Qavgn = 3/2*(vqn*idn-vdn*iqn)
  vq+ : Inport
  vd+ : Inport  Port=2
  iq+ : Inport  Port=3
  id+ : Inport  Port=4
  vq- : Inport  Port=5
  vd- : Inport  Port=6
  iq- : Inport  Port=7
  id- : Inport  Port=8
  Gain : Gain  Gain=3/2
  Gain1 : Gain  Gain=3/2
  Gain2 : Gain  Gain=-1
  Gain3 : Gain  Gain=-1
  Mux{,1..3} (4 alike) : Mux  Inputs=2
  Product{,1..3} (4 alike) : Product
  Sum1 : Sum
  Sum2 : Sum
  Sum8 : Sum
  PQ : Outport
  wires:
  Sum8/1 -> Gain/1
  Gain2/1 -> Mux2/2
  Mux2/1 -> Product2/2
  Product2/1 -> Sum8/2
  Mux/1 -> Product/2
  Product/1 -> Sum8/1
  iq+/1 -> [iqp]
  [iqp] -> Gain2/1, Mux/1
  id+/1 -> [idp]
  [idp] -> Mux2/1, Mux/2
  vq+/1 -> [vqp]
  [vqp] -> Product/1
  vd+/1 -> [vdp]
  [vdp] -> Product2/1
  Gain/1 -> Sum1/1
  Sum1/1 -> PQ/1
  Gain3/1 -> Mux3/2
  Mux1/1 -> Product1/2
  Product3/1 -> Sum2/2
  Product1/1 -> Sum2/1
  [vdn] -> Product3/1
  Mux3/1 -> Product3/2
  [vqn] -> Product1/1
  Sum2/1 -> Gain1/1
  [iqn] -> Gain3/1, Mux1/1
  [idn] -> Mux3/1, Mux1/2
  vq-/1 -> [vqn]
  vd-/1 -> [vdn]
  iq-/1 -> [iqn]
  id-/1 -> [idn]
  Gain1/1 -> Sum1/2

== system Phasor_load/G5/VSC/VSC Control/Control loops/SW, EMT AVG, Phasor Quasi-EMT/Outer-loop/Power calculation ==
  note: AC power calculation using symmetrical components in dq axis
  note: Pavgp = 3/2*(vqp*iqp + vdp*idp) and Qavgp = 3/2*(vqp*idp-vdp*iqp)
  note: P = Pavg + Pc2*cos(2wt) + Ps2*sin(2wt) ---> Pavg = Pavgp + Pavgn
  note: Q = Qavg + Qc2*cos(2wt) + Qs2*sin(2wt) ---> Qavg = Qavgp + Qavgn
  note: Pavgn = 3/2*(vqn*iqn + vdn*idn) and Qavgn = 3/2*(vqn*idn-vdn*iqn)
  vq+ : Inport
  vd+ : Inport  Port=2
  iq+ : Inport  Port=3
  id+ : Inport  Port=4
  vq- : Inport  Port=5
  vd- : Inport  Port=6
  iq- : Inport  Port=7
  id- : Inport  Port=8
  Gain : Gain  Gain=3/2
  Gain1 : Gain  Gain=3/2
  Gain2 : Gain  Gain=-1
  Gain3 : Gain  Gain=-1
  Mux{,1..3} (4 alike) : Mux  Inputs=2
  Product{,1..3} (4 alike) : Product
  Sum1 : Sum
  Sum2 : Sum
  Sum8 : Sum
  PQ : Outport
  wires:
  Sum8/1 -> Gain/1
  Gain2/1 -> Mux2/2
  Mux2/1 -> Product2/2
  Product2/1 -> Sum8/2
  Mux/1 -> Product/2
  Product/1 -> Sum8/1
  iq+/1 -> [iqp]
  [iqp] -> Gain2/1, Mux/1
  id+/1 -> [idp]
  [idp] -> Mux2/1, Mux/2
  vq+/1 -> [vqp]
  [vqp] -> Product/1
  vd+/1 -> [vdp]
  [vdp] -> Product2/1
  Gain/1 -> Sum1/1
  Sum1/1 -> PQ/1
  Gain3/1 -> Mux3/2
  Mux1/1 -> Product1/2
  Product3/1 -> Sum2/2
  Product1/1 -> Sum2/1
  [vdn] -> Product3/1
  Mux3/1 -> Product3/2
  [vqn] -> Product1/1
  Sum2/1 -> Gain1/1
  [iqn] -> Gain3/1, Mux1/1
  [idn] -> Mux3/1, Mux1/2
  vq-/1 -> [vqn]
  vd-/1 -> [vdn]
  iq-/1 -> [iqn]
  id-/1 -> [idn]
  Gain1/1 -> Sum1/2

== system Phasor_load/G5/VSC/VSC Control/Measurements/EMT/PLL aligned with positive-sequence/Notch filter ==
  In : Inport
  Discrete Transfer Fcn : DiscreteTransferFcn  Numerator=[1, -2*cos(theta0), 1]  Denominator="[1, -2*cos(theta0)*r,  r^2]"
  Gain7 : Gain  Gain=Kf
  Out : Outport
  wires:
  Gain7/1 -> Discrete Transfer Fcn/1
  Discrete Transfer Fcn/1 -> Out/1
  In/1 -> Gain7/1

== system Phasor_load/G5/VSC/VSC Control/Measurements/EMT/PLL aligned with positive-sequence/Park transform ==
  note: Park transform (q axis leading)
  abc : Inport
  theta : Inport  Port=2
  0 : Fcn  Expr=1/3*(u(1) + u(2) + u(3))
  Mux2 : Mux  Inputs=2
  Mux3 : Mux  Inputs=3
  d : Fcn  Expr=2/3*(u(1)*sin(u(4)) + u(2)*sin(u(4) - (2*pi)/3) + u(3)*sin(u(4) + (2*pi)/3))
  q : Fcn  Expr=2/3*(u(1)*cos(u(4)) + u(2)*cos(u(4) - (2*pi)/3) + u(3)*cos(u(4) + (2*pi)/3))
  qd0 : Outport  VectorParamsAs1DForOutWhenUnconnected=off
  wires:
  q/1 -> Mux3/1
  Mux2/1 -> q/1, 0/1, d/1
  0/1 -> Mux3/3
  d/1 -> Mux3/2
  theta/1 -> Mux2/2
  abc/1 -> Mux2/1
  Mux3/1 -> qd0/1

== system Phasor_load/G5/VSC/VSC Control/Measurements/EMT/PLL aligned with positive-sequence/Phase-sequence separation ==
  note: Phase-sequence separation based on
      | Delayed Signal Cancellation (DSC) method
  abc : Inport
  Theta : Inport  Port=2
  Complex to Real-Imag1 : ComplexToRealImag
  Complex to Real-Imag2 : ComplexToRealImag
  Complex to Real-Imag3 : ComplexToRealImag
  Constant : Constant  Value=negseq_en
  Demux3 : Demux  Outputs=3
  Exp2 : Math  OutputSignalType=complex
  Exp3 : Math  OutputSignalType=complex
  Gain1 : Gain  Gain=1/2
  Gain4 : Gain  Gain=-1i
  Gain5 : Gain  Gain=1i
  Gain6 : Gain  Gain=1/2
  Gain7 : Gain  Gain=1i
  NOT : Logic  Operator=NOT  IconShape=distinctive  AllPortsSameDT=off  OutDataTypeStr=boolean
  Product3 : Product
  Product4 : Product
  Real-Imag to Complex : RealImagToComplex
  Real-Imag to Complex1 : RealImagToComplex
  Sum1 : Sum  Inputs=|++
  Sum2 : Sum  Inputs=-+|
  Switch : Switch  Criteria=u2 ~= 0  SaturateOnIntegerOverflow=off  InputSameDT=off
  Terminator3 : Terminator
  Transport Delay2 : TransportDelay  DelayTime=1/4*(1/50)
  Transport Delay3 : TransportDelay  DelayTime=1/4*(1/50)
  abc to Alpha-Beta-Zero : powerlib_meascontrol/Transformations/abc to Alpha-Beta-Zero
  q+ : Outport
  d+ : Outport  Port=2
  q- : Outport  Port=3
  d- : Outport  Port=4
  wires:
  NOT/1 -> Switch/2
  Constant/1 -> NOT/1
  Switch/1 -> Product3/1
  Gain6/1 -> Switch/3
  Sum2/1 -> Gain1/1
  Transport Delay2/1 -> Real-Imag to Complex1/1
  Demux3/1 -> Real-Imag to Complex/1
  Complex to Real-Imag1/2 -> Transport Delay3/1
  Gain1/1 -> Product4/2
  Real-Imag to Complex/1 -> Complex to Real-Imag1/1, Sum2/2, Sum1/1, Switch/1
  Complex to Real-Imag3/1 -> d-/1
  Real-Imag to Complex1/1 -> Gain5/1
  Complex to Real-Imag1/1 -> Transport Delay2/1
  Transport Delay3/1 -> Real-Imag to Complex1/2
  Demux3/2 -> Real-Imag to Complex/2
  Product3/1 -> Complex to Real-Imag2/1
  Product4/1 -> Complex to Real-Imag3/1
  abc to Alpha-Beta-Zero/1 -> Demux3/1
  abc/1 -> abc to Alpha-Beta-Zero/1
  Exp3/1 -> Product4/1
  Complex to Real-Imag3/2 -> q-/1
  Complex to Real-Imag2/2 -> q+/1
  Demux3/3 -> Terminator3/1
  Sum1/1 -> Gain6/1
  Gain5/1 -> Sum2/1, Sum1/2
  Exp2/1 -> Product3/2
  Gain4/1 -> Exp2/1
  Theta/1 -> Gain4/1, Gain7/1
  Gain7/1 -> Exp3/1
  Complex to Real-Imag2/1 -> d+/1

== system Phasor_load/G5/VSC/VSC Control/Measurements/EMT/PLL aligned with positive-sequence/Subsystem ==
  note: PI controller with reset port and initial conditions restored after reset or after maximum/minimum values are reached
  in : Inport
  Reset : Inport  Port=2
  Compare To Constant2 : simulink/Logic and Bit Operations/Compare To Constant  relop=~=  const=0  OutDataTypeStr=boolean
  Constant2 : Constant  Value=2*pi*fg
  Gain : Gain  Gain=kp_pll
  Gain1 : Gain  Gain=kp_pll/tau_pll
  Integrator Limited : Integrator  ExternalReset=level  InitialCondition=2*pi*fg  UpperSaturationLimit=10.1*2*pi*fg  LowerSaturationLimit=0.09*2*pi*fg  ShowSaturationPort=on
  Memory1 : Memory
  NOT : Logic  Operator=NOT  IconShape=distinctive  AllPortsSameDT=off  OutDataTypeStr=boolean
  OR2 : Logic  Operator=OR  IconShape=distinctive  AllPortsSameDT=off  OutDataTypeStr=boolean
  Product : Product
  Sum : Sum
  Switch1 : Switch  SaturateOnIntegerOverflow=off  InputSameDT=off
  w : Outport
  wires:
  Switch1/1 -> w/1
  Product/1 -> Gain1/1, Gain/1
  Gain1/1 -> Integrator Limited/1
  Integrator Limited/2 -> Compare To Constant2/1, Switch1/2
  Compare To Constant2/1 -> Memory1/1
  OR2/1 -> Integrator Limited/2, NOT/1
  Constant2/1 -> Switch1/3
  Memory1/1 -> OR2/1
  Reset/1 -> OR2/2
  Gain/1 -> Sum/1
  Integrator Limited/1 -> Sum/2
  Sum/1 -> Switch1/1
  in/1 -> Product/1
  NOT/1 -> Product/2

== system Phasor_load/G5/VSC/VSC Control/Modulation/Phasor I and Phasor PQ/RL time constant/Corrects delay ==
  Clock : Clock
  Gain : Gain  Gain=(2*pi*fg)
  Memory : Memory
  Sum : Sum  Inputs=|+-
  dphi : Outport
  wires:
  Gain/1 -> dphi/1
  Sum/1 -> Gain/1  "Ts"
  Memory/1 -> Sum/2
  Clock/1 -> Sum/1, Memory/1

== system Phasor_load/G6/VSC/VSC Control/Control loops/Phasor I 1st/Outer-loop/Power calculation ==
  note: AC power calculation using symmetrical components in dq axis
  note: Pavgp = 3/2*(vqp*iqp + vdp*idp) and Qavgp = 3/2*(vqp*idp-vdp*iqp)
  note: P = Pavg + Pc2*cos(2wt) + Ps2*sin(2wt) ---> Pavg = Pavgp + Pavgn
  note: Q = Qavg + Qc2*cos(2wt) + Qs2*sin(2wt) ---> Qavg = Qavgp + Qavgn
  note: Pavgn = 3/2*(vqn*iqn + vdn*idn) and Qavgn = 3/2*(vqn*idn-vdn*iqn)
  vq+ : Inport
  vd+ : Inport  Port=2
  iq+ : Inport  Port=3
  id+ : Inport  Port=4
  vq- : Inport  Port=5
  vd- : Inport  Port=6
  iq- : Inport  Port=7
  id- : Inport  Port=8
  Gain : Gain  Gain=3/2
  Gain1 : Gain  Gain=3/2
  Gain2 : Gain  Gain=-1
  Gain3 : Gain  Gain=-1
  Mux{,1..3} (4 alike) : Mux  Inputs=2
  Product{,1..3} (4 alike) : Product
  Sum1 : Sum
  Sum2 : Sum
  Sum8 : Sum
  PQ : Outport
  wires:
  Sum8/1 -> Gain/1
  Gain2/1 -> Mux2/2
  Mux2/1 -> Product2/2
  Product2/1 -> Sum8/2
  Mux/1 -> Product/2
  Product/1 -> Sum8/1
  iq+/1 -> [iqp]
  [iqp] -> Gain2/1, Mux/1
  id+/1 -> [idp]
  [idp] -> Mux2/1, Mux/2
  vq+/1 -> [vqp]
  [vqp] -> Product/1
  vd+/1 -> [vdp]
  [vdp] -> Product2/1
  Gain/1 -> Sum1/1
  Sum1/1 -> PQ/1
  Gain3/1 -> Mux3/2
  Mux1/1 -> Product1/2
  Product3/1 -> Sum2/2
  Product1/1 -> Sum2/1
  [vdn] -> Product3/1
  Mux3/1 -> Product3/2
  [vqn] -> Product1/1
  Sum2/1 -> Gain1/1
  [iqn] -> Gain3/1, Mux1/1
  [idn] -> Mux3/1, Mux1/2
  vq-/1 -> [vqn]
  vd-/1 -> [vdn]
  iq-/1 -> [iqn]
  id-/1 -> [idn]
  Gain1/1 -> Sum1/2

== system Phasor_load/G6/VSC/VSC Control/Control loops/Phasor I ref/Outer-loop/Power calculation ==
  note: Pavgn = 3/2*(vqn*iqn + vdn*idn) and Qavgn = 3/2*(vqn*idn-vdn*iqn)
  note: Q = Qavg + Qc2*cos(2wt) + Qs2*sin(2wt) ---> Qavg = Qavgp + Qavgn
  note: P = Pavg + Pc2*cos(2wt) + Ps2*sin(2wt) ---> Pavg = Pavgp + Pavgn
  note: Pavgp = 3/2*(vqp*iqp + vdp*idp) and Qavgp = 3/2*(vqp*idp-vdp*iqp)
  note: AC power calculation using symmetrical components in dq axis
  vq+ : Inport
  vd+ : Inport  Port=2
  iq+ : Inport  Port=3
  id+ : Inport  Port=4
  vq- : Inport  Port=5
  vd- : Inport  Port=6
  iq- : Inport  Port=7
  id- : Inport  Port=8
  Gain : Gain  Gain=3/2
  Gain1 : Gain  Gain=3/2
  Gain2 : Gain  Gain=-1
  Gain3 : Gain  Gain=-1
  Mux{,1..3} (4 alike) : Mux  Inputs=2
  Product{,1..3} (4 alike) : Product
  Sum1 : Sum
  Sum2 : Sum
  Sum8 : Sum
  PQ : Outport
  wires:
  Gain1/1 -> Sum1/2
  id-/1 -> [idn]
  iq-/1 -> [iqn]
  vd-/1 -> [vdn]
  vq-/1 -> [vqn]
  [idn] -> Mux1/2, Mux3/1
  [iqn] -> Mux1/1, Gain3/1
  Sum2/1 -> Gain1/1
  [vqn] -> Product1/1
  Mux3/1 -> Product3/2
  [vdn] -> Product3/1
  Product1/1 -> Sum2/1
  Product3/1 -> Sum2/2
  Mux1/1 -> Product1/2
  Gain3/1 -> Mux3/2
  Sum1/1 -> PQ/1
  Gain/1 -> Sum1/1
  [vdp] -> Product2/1
  vd+/1 -> [vdp]
  [vqp] -> Product/1
  vq+/1 -> [vqp]
  [idp] -> Mux/2, Mux2/1
  id+/1 -> [idp]
  [iqp] -> Mux/1, Gain2/1
  iq+/1 -> [iqp]
  Product/1 -> Sum8/1
  Mux/1 -> Product/2
  Product2/1 -> Sum8/2
  Mux2/1 -> Product2/2
  Gain2/1 -> Mux2/2
  Sum8/1 -> Gain/1

== system Phasor_load/G6/VSC/VSC Control/Control loops/Phasor PQ 1st/Outer-loop/Power calculation ==
  note: AC power calculation using symmetrical components in dq axis
  note: Pavgp = 3/2*(vqp*iqp + vdp*idp) and Qavgp = 3/2*(vqp*idp-vdp*iqp)
  note: P = Pavg + Pc2*cos(2wt) + Ps2*sin(2wt) ---> Pavg = Pavgp + Pavgn
  note: Q = Qavg + Qc2*cos(2wt) + Qs2*sin(2wt) ---> Qavg = Qavgp + Qavgn
  note: Pavgn = 3/2*(vqn*iqn + vdn*idn) and Qavgn = 3/2*(vqn*idn-vdn*iqn)
  vq+ : Inport
  vd+ : Inport  Port=2
  iq+ : Inport  Port=3
  id+ : Inport  Port=4
  vq- : Inport  Port=5
  vd- : Inport  Port=6
  iq- : Inport  Port=7
  id- : Inport  Port=8
  Gain : Gain  Gain=3/2
  Gain1 : Gain  Gain=3/2
  Gain2 : Gain  Gain=-1
  Gain3 : Gain  Gain=-1
  Mux{,1..3} (4 alike) : Mux  Inputs=2
  Product{,1..3} (4 alike) : Product
  Sum1 : Sum
  Sum2 : Sum
  Sum8 : Sum
  PQ : Outport
  wires:
  Sum8/1 -> Gain/1
  Gain2/1 -> Mux2/2
  Mux2/1 -> Product2/2
  Product2/1 -> Sum8/2
  Mux/1 -> Product/2
  Product/1 -> Sum8/1
  iq+/1 -> [iqp]
  [iqp] -> Gain2/1, Mux/1
  id+/1 -> [idp]
  [idp] -> Mux2/1, Mux/2
  vq+/1 -> [vqp]
  [vqp] -> Product/1
  vd+/1 -> [vdp]
  [vdp] -> Product2/1
  Gain/1 -> Sum1/1
  Sum1/1 -> PQ/1
  Gain3/1 -> Mux3/2
  Mux1/1 -> Product1/2
  Product3/1 -> Sum2/2
  Product1/1 -> Sum2/1
  [vdn] -> Product3/1
  Mux3/1 -> Product3/2
  [vqn] -> Product1/1
  Sum2/1 -> Gain1/1
  [iqn] -> Gain3/1, Mux1/1
  [idn] -> Mux3/1, Mux1/2
  vq-/1 -> [vqn]
  vd-/1 -> [vdn]
  iq-/1 -> [iqn]
  id-/1 -> [idn]
  Gain1/1 -> Sum1/2

== system Phasor_load/G6/VSC/VSC Control/Control loops/SW, EMT AVG, Phasor Quasi-EMT/Outer-loop/Power calculation ==
  note: AC power calculation using symmetrical components in dq axis
  note: Pavgp = 3/2*(vqp*iqp + vdp*idp) and Qavgp = 3/2*(vqp*idp-vdp*iqp)
  note: P = Pavg + Pc2*cos(2wt) + Ps2*sin(2wt) ---> Pavg = Pavgp + Pavgn
  note: Q = Qavg + Qc2*cos(2wt) + Qs2*sin(2wt) ---> Qavg = Qavgp + Qavgn
  note: Pavgn = 3/2*(vqn*iqn + vdn*idn) and Qavgn = 3/2*(vqn*idn-vdn*iqn)
  vq+ : Inport
  vd+ : Inport  Port=2
  iq+ : Inport  Port=3
  id+ : Inport  Port=4
  vq- : Inport  Port=5
  vd- : Inport  Port=6
  iq- : Inport  Port=7
  id- : Inport  Port=8
  Gain : Gain  Gain=3/2
  Gain1 : Gain  Gain=3/2
  Gain2 : Gain  Gain=-1
  Gain3 : Gain  Gain=-1
  Mux{,1..3} (4 alike) : Mux  Inputs=2
  Product{,1..3} (4 alike) : Product
  Sum1 : Sum
  Sum2 : Sum
  Sum8 : Sum
  PQ : Outport
  wires:
  Sum8/1 -> Gain/1
  Gain2/1 -> Mux2/2
  Mux2/1 -> Product2/2
  Product2/1 -> Sum8/2
  Mux/1 -> Product/2
  Product/1 -> Sum8/1
  iq+/1 -> [iqp]
  [iqp] -> Gain2/1, Mux/1
  id+/1 -> [idp]
  [idp] -> Mux2/1, Mux/2
  vq+/1 -> [vqp]
  [vqp] -> Product/1
  vd+/1 -> [vdp]
  [vdp] -> Product2/1
  Gain/1 -> Sum1/1
  Sum1/1 -> PQ/1
  Gain3/1 -> Mux3/2
  Mux1/1 -> Product1/2
  Product3/1 -> Sum2/2
  Product1/1 -> Sum2/1
  [vdn] -> Product3/1
  Mux3/1 -> Product3/2
  [vqn] -> Product1/1
  Sum2/1 -> Gain1/1
  [iqn] -> Gain3/1, Mux1/1
  [idn] -> Mux3/1, Mux1/2
  vq-/1 -> [vqn]
  vd-/1 -> [vdn]
  iq-/1 -> [iqn]
  id-/1 -> [idn]
  Gain1/1 -> Sum1/2

== system Phasor_load/G6/VSC/VSC Control/Measurements/EMT/PLL aligned with positive-sequence/Notch filter ==
  In : Inport
  Discrete Transfer Fcn : DiscreteTransferFcn  Numerator=[1, -2*cos(theta0), 1]  Denominator="[1, -2*cos(theta0)*r,  r^2]"
  Gain7 : Gain  Gain=Kf
  Out : Outport
  wires:
  Gain7/1 -> Discrete Transfer Fcn/1
  Discrete Transfer Fcn/1 -> Out/1
  In/1 -> Gain7/1

== system Phasor_load/G6/VSC/VSC Control/Measurements/EMT/PLL aligned with positive-sequence/Park transform ==
  note: Park transform (q axis leading)
  abc : Inport
  theta : Inport  Port=2
  0 : Fcn  Expr=1/3*(u(1) + u(2) + u(3))
  Mux2 : Mux  Inputs=2
  Mux3 : Mux  Inputs=3
  d : Fcn  Expr=2/3*(u(1)*sin(u(4)) + u(2)*sin(u(4) - (2*pi)/3) + u(3)*sin(u(4) + (2*pi)/3))
  q : Fcn  Expr=2/3*(u(1)*cos(u(4)) + u(2)*cos(u(4) - (2*pi)/3) + u(3)*cos(u(4) + (2*pi)/3))
  qd0 : Outport  VectorParamsAs1DForOutWhenUnconnected=off
  wires:
  q/1 -> Mux3/1
  Mux2/1 -> q/1, 0/1, d/1
  0/1 -> Mux3/3
  d/1 -> Mux3/2
  theta/1 -> Mux2/2
  abc/1 -> Mux2/1
  Mux3/1 -> qd0/1
